simulink model "test_rectifiers"  (R2025b)
settings: Solver=VariableStepAuto  StartTime=0.0  StopTime=5/60  RelTol=1e-3
undefined symbols (not defined in the file): DiscIntNeverNeededParam
libraries: ee_lib_for_power_systems x15, fl_lib x10, nesl_utility x5, ee_lib x5, eeThyristorSixPulseGenerator x3
settings Model: Creator=gdudgeon  LastModifiedBy=gdudgeon
settings RTWCC: GPUComputeCapability=3.5

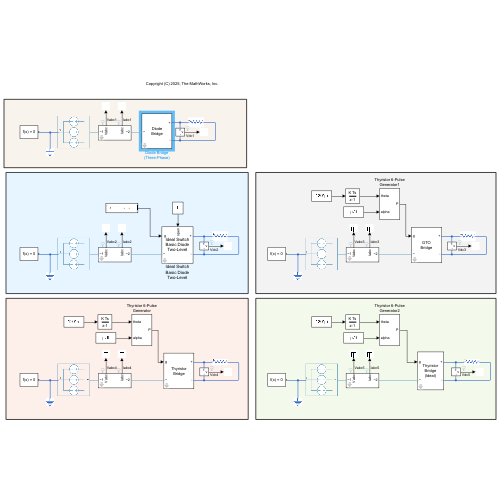
[thumbnail: Simulink's stored preview of the top-level diagram]
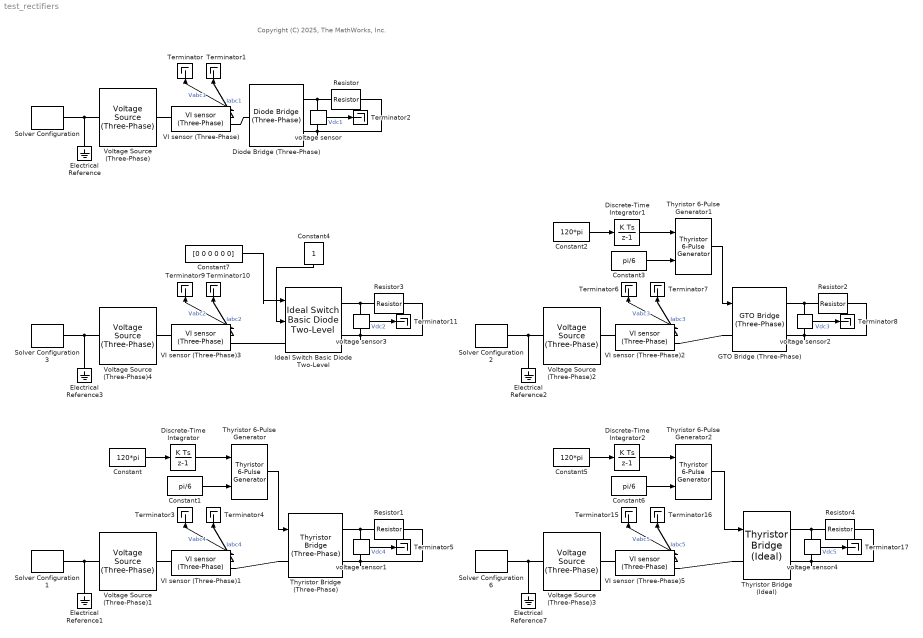
== system test_rectifiers ==
  note: Copyright (C) 2025, The MathWorks, Inc.
  Constant : Constant  Value=120*pi  SampleTime=-1
  Constant1 : Constant  Value=pi/6  SampleTime=-1
  Constant2 : Constant  Value=120*pi  SampleTime=-1
  Constant3 : Constant  Value=pi/6  SampleTime=-1
  Constant4 : Constant  SampleTime=-1
  Constant5 : Constant  Value=120*pi  SampleTime=-1
  Constant6 : Constant  Value=pi/6  SampleTime=-1
  Constant7 : Constant  Value=[0 0 0 0 0 0]  SampleTime=-1
  Diode Bridge (Three-Phase) : ee_lib_for_power_systems/Power Converters/Diode Bridge (Three-Phase)  Vf=1e-3  Ron=1e-3  Goff=1e-5
      settings: SourceProductName=Support Library for Power Systems
  Discrete-Time Integrator : DiscreteIntegrator  SampleTime=-1  ICPrevOutput=DiscIntNeverNeededParam  ICPrevScaledInput=DiscIntNeverNeededParam
  Discrete-Time Integrator1 : DiscreteIntegrator  SampleTime=-1  ICPrevOutput=DiscIntNeverNeededParam  ICPrevScaledInput=DiscIntNeverNeededParam
  Discrete-Time Integrator2 : DiscreteIntegrator  SampleTime=-1  ICPrevOutput=DiscIntNeverNeededParam  ICPrevScaledInput=DiscIntNeverNeededParam
  Electrical Reference{,1..3,7} (5 alike) : fl_lib/Electrical/Electrical Elements/Electrical Reference
  GTO Bridge (Three-Phase) : ee_lib_for_power_systems/Power Converters/GTO Bridge (Three-Phase)  Ron=1e-5  Goff=1e-5  Vfs=1e-3  Vfd=1e-3  run_time=off
      settings: SourceProductName=Support Library for Power Systems
  Ideal Switch Basic Diode Two-Level : ee_lib_for_power_systems/Power Converters/Ideal Switch Basic Diode Two-Level  Ron=1e-3  Goff=1e-5
      settings: SourceProductName=Support Library for Power Systems
  Resistor{,1..4} (5 alike) : fl_lib/Electrical/Electrical Elements/Resistor  R=1 Ohm  i_specify=off  i_priority=None  i=0 A  i_nominal_specify=off  i_nominal_value=1  i_nominal_unit=A  v_specify=off  v_priority=None  v=0 V  v_nominal_specify=off  v_nominal_value=1  v_nominal_unit=V
  Solver Configuration {,1..3} (4 alike) : nesl_utility/Solver Configuration  PhysicalDomain=network_engine_domain  SubClassName=solver  LeftPortType=input  RightPortType=generic  Tones=[]  Harmonics=[]  SimulateNoise=off  Profile=off  UseLocalSampling=off  EnableSwitchedLinearOptims=on  FrequencyDomain=off  UseCCode=off  RelTol=0.001  AbsTol=0.001  MinStep=1e-09  ToWorkspace=off  RevertToSquareIcSolve=off  NumHomotopyIterations=100  PhasorMode=off  PhasorModeNumHarmonics=1  ConsistencySolver=NEWTON_XTOL_AFTER_FTOL  IndexReductionMethod=None  DoDC=off  ResidualTolerance=1e-09  ConsistencyTolSource=GLOBAL  ConsistencyAbsTol=0.001  ConsistencyRelTol=0.001  ConsistencyTolFactor=0.001  UseLocalSolver=on  LocalSolverChoice=NE_BACKWARD_EULER_ADVANCER  ResolveIndetEquations=off  FunctionEvalNumThread=1  LocalSolverSampleTime=50e-6  DoFixedCost=on  MaxNonlinIter=2  MaxModeIter=2  ComputeImpulses=off  ImpulseIterations=2  LinearAlgebra=Sparse  LinearAlgebraNumThread=0  EquationFormulation=NE_TIME_EF  DelaysMemoryBudget=1024  AutomaticFiltering=off  FilteringTimeConstant=0.001  PartitionStorageMethod=AS_NEEDED  PartitionMemoryBudget=1024  PartitionMethod=ROBUST  MultibodyUseLocalSolver=off  MultibodyLocalSolverChoice=ODE1  MultibodyLocalSolverSampleTime=0.001
  Solver Configuration 6 : nesl_utility/Solver Configuration  PhysicalDomain=network_engine_domain  SubClassName=solver  LeftPortType=input  RightPortType=generic  Tones=[]  Harmonics=[]  SimulateNoise=off  Profile=off  UseLocalSampling=off  EnableSwitchedLinearOptims=on  FrequencyDomain=off  UseCCode=off  RelTol=0.001  AbsTol=0.001  MinStep=1e-09  ToWorkspace=off  RevertToSquareIcSolve=off  NumHomotopyIterations=100  PhasorMode=off  PhasorModeNumHarmonics=1  ConsistencySolver=NEWTON_XTOL_AFTER_FTOL  IndexReductionMethod=None  DoDC=off  ResidualTolerance=1e-09  ConsistencyTolSource=GLOBAL  ConsistencyAbsTol=0.001  ConsistencyRelTol=0.001  ConsistencyTolFactor=0.001  UseLocalSolver=on  LocalSolverChoice=NE_PARTITIONING_ADVANCER  ResolveIndetEquations=off  FunctionEvalNumThread=1  LocalSolverSampleTime=50e-6  DoFixedCost=off  MaxNonlinIter=2  MaxModeIter=2  ComputeImpulses=off  ImpulseIterations=2  LinearAlgebra=Sparse  LinearAlgebraNumThread=0  EquationFormulation=NE_TIME_EF  DelaysMemoryBudget=1024  AutomaticFiltering=off  FilteringTimeConstant=0.001  PartitionStorageMethod=AS_NEEDED  PartitionMemoryBudget=1024  PartitionMethod=ROBUST  MultibodyUseLocalSolver=off  MultibodyLocalSolverChoice=ODE1  MultibodyLocalSolverSampleTime=0.001
  Terminator{,1..11,15..17} (15 alike) : Terminator
  Thyristor 6-Pulse Generator : eeThyristorSixPulseGenerator/Thyristor 6-Pulse Generator  Ord=Natural order of commutation  Pw=5*pi/6  Ts=5e-5
      settings: LibrarySourceBlock=|
      | ee_sl_lib/Pulse Width
      | Modulation/Thyristor 6-Pulse
      | Generator
  Thyristor 6-Pulse Generator1 : eeThyristorSixPulseGenerator/Thyristor 6-Pulse Generator  Ord=Natural order of commutation  Pw=5*pi/6  Ts=5e-5
      settings: LibrarySourceBlock=|
      | ee_sl_lib/Pulse Width
      | Modulation/Thyristor 6-Pulse
      | Generator
  Thyristor 6-Pulse Generator2 : eeThyristorSixPulseGenerator/Thyristor 6-Pulse Generator  Ord=Natural order of commutation  Pw=5*pi/6  Ts=5e-5
      settings: LibrarySourceBlock=|
      | ee_sl_lib/Pulse Width
      | Modulation/Thyristor 6-Pulse
      | Generator
  Thyristor Bridge (Ideal) : ee_lib_for_power_systems/Power Converters/Thyristor Bridge (Ideal)  Ron=1e-5  Goff=1e-5  Vf=1e-3
      settings: SourceProductName=Support Library for Power Systems
  Thyristor Bridge (Three-Phase) : ee_lib_for_power_systems/Power Converters/Thyristor Bridge (Three-Phase)  Ron=1e-5  Goff=1e-5  Vfs=1e-3  run_time=off
      settings: SourceProductName=Support Library for Power Systems
  VI sensor (Three-Phase){,1..3,5} (5 alike) : ee_lib_for_power_systems/Sense and Measure/VI sensor (Three-Phase)  volt_meas=Line-to-Line (Line Voltage)  meas_units=SI  Vnom=24e3  Pnom=100e6
      settings: SourceProductName=Support Library for Power Systems
  Voltage Source (Three-Phase){,1..4} (5 alike) : ee_lib/Sources/Voltage Source (Three-Phase)  vline_rms=sqrt(3) * 100 / sqrt(2) V  shift=0 deg  freq=60 Hz  impedance_option=1  SShortCircuit=1e6 A*V  XR=15  R=0.01 Ohm  L=3.97e-4 H  harmonic_option=0  harmonic_orders=[5, 7, 11, 13]  harmonic_ratios=[.1, .1, .1, .1]  G_parasitic=0 1/Ohm  I_specify=off  I_priority=None  I=[0, 0, 0] A  I_nominal_specify=off  I_nominal_value=1  I_nominal_unit=A
  voltage sensor{,1..4} (5 alike) : ee_lib_for_power_systems/Sense and Measure/voltage sensor  SystemSampleTime=-1  VariantActivationTime=update diagram  EmptyChoice=off  PassThrough=off  PassThroughVariantControl=(default)  EmptyChoiceVariantControl=(default)  AllowFlexibleInterface=on  Latency=0  AutoFrameSizeCalculation=off
      settings: SourceProductName=Support Library for Power Systems  PortSchema="{\"entries\":[{\"content\":{\"sides\":[{\"content\":{},\"type\":\"ConnectorPlacement.EquallySpacedRectSide\",\"uuid\":\"799648ba-196f-427a-9565-f64fffdae700\"},{\"content\":{\"connectorIds\":[\"Out1\"],\"side\":\"RIGHT\"},\"type\":\"ConnectorPlacement.EquallySpacedRectSide\",\"uuid\":\"662de5d5-c2ef-406c-9235-94a35f9d89fb\"},{\"content\":{\"connectorIds\":[\"LConn1\"],\"side\":\"TOP\"},\"type\":\"ConnectorPlacement.EquallySpacedRectSide\",\"uuid\":\"67dc8fec-98bd-426f-bbe6-5723f2587b12\"},{\"content\":{\"connectorIds\":[\"RConn1\"],\"side\":\"BOTTOM\"},\"type\":\"ConnectorPlacement.EquallySpacedRectSide\",\"uuid\":\"7e3d7354-1ab6-44d8-9b44-c988118d052c\"}]},\"type\":\"ConnectorPlacement.EquallySpacedConnector\",\"uuid\":\"3e33dbb3-529a-4788-9727-18d62c402281\"}],\"packageUris\":[\"http://schema.mathworks.com/mf0/Connector/R2020b\"],\"version\":\"1.0\"}"
  wires:
  VI sensor (Three-Phase)/1 -> Terminator/1  "Vabc1"
  VI sensor (Three-Phase)/2 -> Terminator1/1  "Iabc1"
  voltage sensor/1 -> Terminator2/1  "Vdc1"
  voltage sensor1/1 -> Terminator5/1  "Vdc4"
  VI sensor (Three-Phase)1/2 -> Terminator4/1  "Iabc4"
  VI sensor (Three-Phase)1/1 -> Terminator3/1  "Vabc4"
  Thyristor 6-Pulse Generator/1 -> Thyristor Bridge (Three-Phase)/1
  Discrete-Time Integrator/1 -> Thyristor 6-Pulse Generator/1
  Constant/1 -> Discrete-Time Integrator/1
  Constant1/1 -> Thyristor 6-Pulse Generator/2
  Constant3/1 -> Thyristor 6-Pulse Generator1/2
  Constant2/1 -> Discrete-Time Integrator1/1
  Discrete-Time Integrator1/1 -> Thyristor 6-Pulse Generator1/1
  Thyristor 6-Pulse Generator1/1 -> GTO Bridge (Three-Phase)/1
  VI sensor (Three-Phase)2/1 -> Terminator6/1  "Vabc3"
  VI sensor (Three-Phase)2/2 -> Terminator7/1  "Iabc3"
  voltage sensor2/1 -> Terminator8/1  "Vdc3"
  voltage sensor4/1 -> Terminator17/1  "Vdc5"
  VI sensor (Three-Phase)5/2 -> Terminator16/1  "Iabc5"
  VI sensor (Three-Phase)5/1 -> Terminator15/1  "Vabc5"
  Thyristor 6-Pulse Generator2/1 -> Thyristor Bridge (Ideal)/1
  Discrete-Time Integrator2/1 -> Thyristor 6-Pulse Generator2/1
  Constant5/1 -> Discrete-Time Integrator2/1
  Constant6/1 -> Thyristor 6-Pulse Generator2/2
  VI sensor (Three-Phase)3/1 -> Terminator9/1  "Vabc2"
  VI sensor (Three-Phase)3/2 -> Terminator10/1  "Iabc2"
  voltage sensor3/1 -> Terminator11/1  "Vdc2"
  Constant4/1 -> Ideal Switch Basic Diode Two-Level/2
  Constant7/1 -> Ideal Switch Basic Diode Two-Level/1
  connections:
  "Solver Configuration "/RConn1 -- Electrical Reference/LConn1 -- Voltage Source (Three-Phase)/LConn1
  Resistor/LConn1 -- voltage sensor/LConn1 -- Diode Bridge (Three-Phase)/RConn1
  VI sensor (Three-Phase)/LConn1 -- Voltage Source (Three-Phase)/RConn1
  VI sensor (Three-Phase)/RConn1 -- Diode Bridge (Three-Phase)/LConn1
  Solver Configuration 1/RConn1 -- Voltage Source (Three-Phase)1/LConn1 -- Electrical Reference1/LConn1
  voltage sensor1/RConn1 -- Thyristor Bridge (Three-Phase)/RConn2 -- Resistor1/RConn1
  voltage sensor1/LConn1 -- Thyristor Bridge (Three-Phase)/RConn1 -- Resistor1/LConn1
  Thyristor Bridge (Three-Phase)/LConn1 -- VI sensor (Three-Phase)1/RConn1
  VI sensor (Three-Phase)1/LConn1 -- Voltage Source (Three-Phase)1/RConn1
  Diode Bridge (Three-Phase)/RConn2 -- Resistor/RConn1 -- voltage sensor/RConn1
  Voltage Source (Three-Phase)2/LConn1 -- Solver Configuration 2/RConn1 -- Electrical Reference2/LConn1
  Resistor2/RConn1 -- GTO Bridge (Three-Phase)/RConn2 -- voltage sensor2/RConn1
  Resistor2/LConn1 -- GTO Bridge (Three-Phase)/RConn1 -- voltage sensor2/LConn1
  GTO Bridge (Three-Phase)/LConn1 -- VI sensor (Three-Phase)2/RConn1
  VI sensor (Three-Phase)2/LConn1 -- Voltage Source (Three-Phase)2/RConn1
  Voltage Source (Three-Phase)3/LConn1 -- Electrical Reference7/LConn1 -- Solver Configuration 6/RConn1
  voltage sensor4/RConn1 -- Thyristor Bridge (Ideal)/RConn2 -- Resistor4/RConn1
  voltage sensor4/LConn1 -- Thyristor Bridge (Ideal)/RConn1 -- Resistor4/LConn1
  VI sensor (Three-Phase)5/LConn1 -- Voltage Source (Three-Phase)3/RConn1
  Thyristor Bridge (Ideal)/LConn1 -- VI sensor (Three-Phase)5/RConn1
  Solver Configuration 3/RConn1 -- Electrical Reference3/LConn1 -- Voltage Source (Three-Phase)4/LConn1
  voltage sensor3/RConn1 -- Ideal Switch Basic Diode Two-Level/RConn2 -- Resistor3/RConn1
  voltage sensor3/LConn1 -- Ideal Switch Basic Diode Two-Level/RConn1 -- Resistor3/LConn1
  VI sensor (Three-Phase)3/LConn1 -- Voltage Source (Three-Phase)4/RConn1
  Ideal Switch Basic Diode Two-Level/LConn1 -- VI sensor (Three-Phase)3/RConn1
